simulink model "asdsl"  (R2014a)
settings: Solver=ode45  StartTime=0.0  StopTime=10.0  RelTol=1e-3
undefined symbols (not defined in the file): sf
libraries: commdigbbndpm3 x7, commseqgen2 x4, commchan3 x2, commrandsrc2 x2, dspsigops x2, commfilt2 x2, commsink2 x1
settings Model: Creator=QC  LastModifiedBy=QC

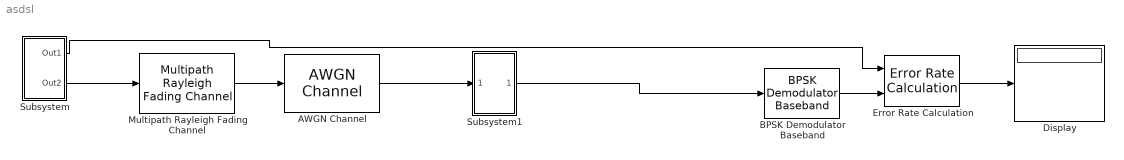
== system asdsl ==
  AWGN Channel : commchan3/AWGN Channel  InputProcessing=Columns as channels (frame based)  seed=67  noiseMode="Signal to noise ratio  (SNR)"  EbNodB=10  EsNodB=10  SNRdB=10  bitsPerSym=1  Ps=1  Tsym=1  variance=1
  BPSK Demodulator Baseband : commdigbbndpm3/BPSK Demodulator Baseband  Ph=0  DecType=Hard decision  VarSource=Dialog  Variance=1  outDtype=Inherit via internal rule  derotateFactorWordLen=16
  Display : Display
  Error Rate Calculation : commsink2/Error Rate Calculation  N=0  st_delay=0  cp_mode=Entire frame  subframe=[]  PMode=Port  WsName=ErrorVec  RsMode2=off  stop=off  numErr=100  maxBits=1e6
  Multipath Rayleigh Fading Channel : commchan3/Multipath Rayleigh Fading Channel  maxDopplerShift=40  spectrumType=Jakes  sigmaGaussian=1/sqrt(2)  coeffRounded=[1 -1.72 0.785]  freqMinMaxRJakes=[0 1]  freqMinMaxAJakes=[0 1]  sigmaGaussian1=1/sqrt(2)  sigmaGaussian2=1/sqrt(2)  centerFreqGaussian1=0.0  centerFreqGaussian2=0.0  gainGaussian1=0.5  gainGaussian2=0.5  coeffBell=9  dopplerSpectrum=doppler.jakes  pathDelays=[0]  avgPathGaindB=[0]  normalizePathGains=on  seed=73  enableProbe=0  openVisAtStart=off  outPathGains=off  outDelay=off
  Subsystem : Subsystem
  Subsystem1 : Subsystem
  wires:
  BPSK Demodulator Baseband/1 -> Error Rate Calculation/2
  Error Rate Calculation/1 -> Display/1
  Subsystem/1(Out1) -> Error Rate Calculation/1
  Subsystem/2(Out2) -> Multipath Rayleigh Fading Channel/1
  AWGN Channel/1 -> Subsystem1/1(In1)
  Subsystem1/1(Out1) -> BPSK Demodulator Baseband/1
  Multipath Rayleigh Fading Channel/1 -> AWGN Channel/1

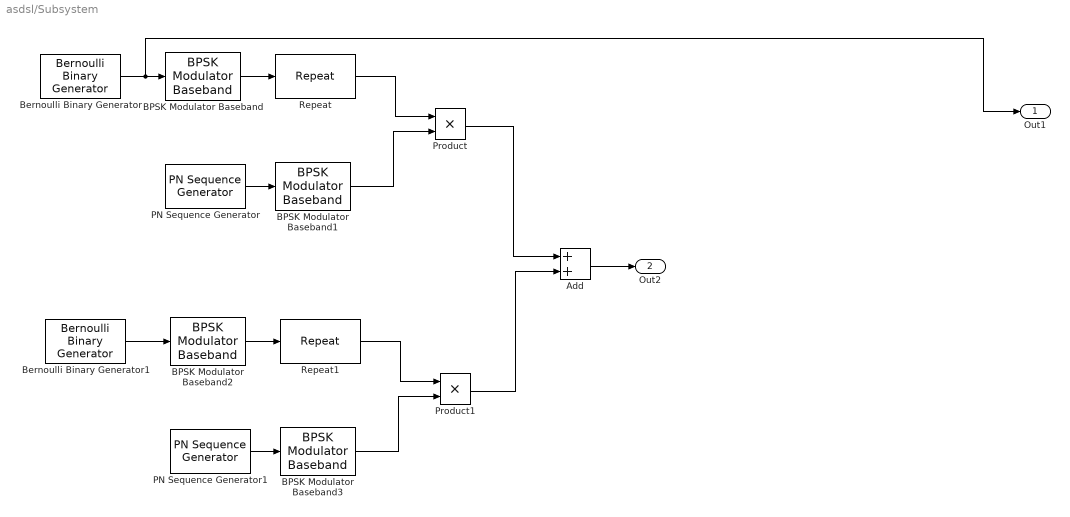
== system asdsl/Subsystem ==
  Add : Sum
  BPSK Modulator Baseband{,1..3} (4 alike) : commdigbbndpm3/BPSK Modulator Baseband  Ph=0  outDtype=double  outWordLen=16  outUDDataType=sfix(16)  outFracLenMode=Best precision  outFracLen=15
  Bernoulli Binary Generator : commrandsrc2/Bernoulli Binary Generator  P=0.5  seed=61  Ts=sf/3.84e6  frameBased=on  sampPerFrame=10  orient=off  outDataType=double
  Bernoulli Binary Generator1 : commrandsrc2/Bernoulli Binary Generator  P=1  seed=61  Ts=sf/3.84e6  frameBased=on  sampPerFrame=10  orient=off  outDataType=double
  PN Sequence Generator : commseqgen2/PN Sequence Generator  poly=[1 0 0 0 0 1 1]  ini_sta=[0 0 0 0 0 1]  outBitMaskSource=Dialog parameter  shift=0  outVarSiz=off  maxOutSizeMode=Dialog parameter  maxOutSize=[10 1]  Ts=1/3.84e6  frameBased=on  sampPerFrame=sf*10  reset=off  bitPackedOutputs=off  outDataType=double  numPackedBits=8  bitPackDataSigned=off  bitPackedOutDType=double
  PN Sequence Generator1 : commseqgen2/PN Sequence Generator  poly=[1 0 0 0 0 1 1]  ini_sta=[0 0 1 0 1 1]  outBitMaskSource=Dialog parameter  shift=0  outVarSiz=off  maxOutSizeMode=Dialog parameter  maxOutSize=[10 1]  Ts=1/3.84e6  frameBased=on  sampPerFrame=sf*10  reset=off  bitPackedOutputs=off  outDataType=double  numPackedBits=8  bitPackDataSigned=off  bitPackedOutDType=double
  Product : Product
  Product1 : Product
  Repeat : dspsigops/Repeat  N=sf  InputProcessing=Columns as channels (frame based)  RateOptions=Enforce single-rate processing  ic=0  mode=Unused parameter value
  Repeat1 : dspsigops/Repeat  N=sf  InputProcessing=Columns as channels (frame based)  RateOptions=Enforce single-rate processing  ic=0  mode=Unused parameter value
  Out1 : Outport
  Out2 : Outport  Port=2
  wires:
  PN Sequence Generator/1 -> BPSK Modulator Baseband1/1
  BPSK Modulator Baseband1/1 -> Product/2
  Repeat/1 -> Product/1
  Bernoulli Binary Generator/1 -> Out1/1, BPSK Modulator Baseband/1
  BPSK Modulator Baseband/1 -> Repeat/1
  PN Sequence Generator1/1 -> BPSK Modulator Baseband3/1
  BPSK Modulator Baseband3/1 -> Product1/2
  Repeat1/1 -> Product1/1
  Bernoulli Binary Generator1/1 -> BPSK Modulator Baseband2/1
  BPSK Modulator Baseband2/1 -> Repeat1/1
  Add/1 -> Out2/1
  Product/1 -> Add/1
  Product1/1 -> Add/2

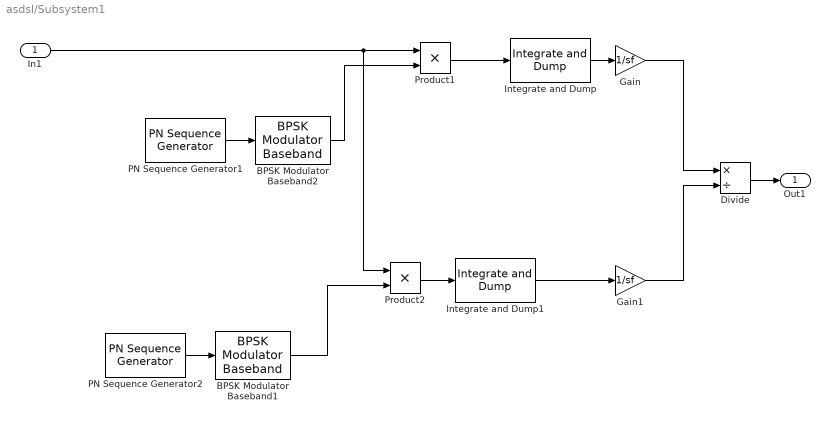
== system asdsl/Subsystem1 ==
  In1 : Inport
  BPSK Modulator Baseband1 : commdigbbndpm3/BPSK Modulator Baseband  Ph=0  outDtype=double  outWordLen=16  outUDDataType=sfix(16)  outFracLenMode=Best precision  outFracLen=15
  BPSK Modulator Baseband2 : commdigbbndpm3/BPSK Modulator Baseband  Ph=0  outDtype=double  outWordLen=16  outUDDataType=sfix(16)  outFracLenMode=Best precision  outFracLen=15
  Divide : Product  Inputs=*/
  Gain : Gain  Gain=1/sf
  Gain1 : Gain  Gain=1/sf
  Integrate and Dump : commfilt2/Integrate and Dump  obssamples=sf  offsetsamples=0  nodump=off  roundingMode=Floor  overflowMode=off
  Integrate and Dump1 : commfilt2/Integrate and Dump  obssamples=sf  offsetsamples=0  nodump=off  roundingMode=Floor  overflowMode=off
  PN Sequence Generator1 : commseqgen2/PN Sequence Generator  poly=[1 0 0 0 0 1 1]  ini_sta=[0 0 0 0 0 1]  outBitMaskSource=Dialog parameter  shift=0  outVarSiz=off  maxOutSizeMode=Dialog parameter  maxOutSize=[10 1]  Ts=1/3.84e6  frameBased=on  sampPerFrame=sf*10  reset=off  bitPackedOutputs=off  outDataType=double  numPackedBits=8  bitPackDataSigned=off  bitPackedOutDType=double
  PN Sequence Generator2 : commseqgen2/PN Sequence Generator  poly=[1 0 0 0 0 1 1]  ini_sta=[0 0 1 0 1 1]  outBitMaskSource=Dialog parameter  shift=0  outVarSiz=off  maxOutSizeMode=Dialog parameter  maxOutSize=[10 1]  Ts=1/3.84e6  frameBased=on  sampPerFrame=sf*10  reset=off  bitPackedOutputs=off  outDataType=double  numPackedBits=8  bitPackDataSigned=off  bitPackedOutDType=double
  Product1 : Product
  Product2 : Product
  Out1 : Outport
  wires:
  Product1/1 -> Integrate and Dump/1
  BPSK Modulator Baseband2/1 -> Product1/2
  In1/1 -> Product2/1, Product1/1
  Integrate and Dump/1 -> Gain/1
  PN Sequence Generator1/1 -> BPSK Modulator Baseband2/1
  PN Sequence Generator2/1 -> BPSK Modulator Baseband1/1
  BPSK Modulator Baseband1/1 -> Product2/2
  Integrate and Dump1/1 -> Gain1/1
  Product2/1 -> Integrate and Dump1/1
  Gain/1 -> Divide/1
  Gain1/1 -> Divide/2
  Divide/1 -> Out1/1
